simulink model "sampleModel103"  (R2023a)
settings: Solver=VariableStepAuto  StartTime=0.0  StopTime=10.0  RelTol=1e-3
undefined symbols (not defined in the file): DiscIntNeverNeededParam, Newton, Raphson
libraries: simulink x49, slpidlib x14
(part 1 of 3)
settings Model: Creator=TSMC  LastModifiedBy=TSMC

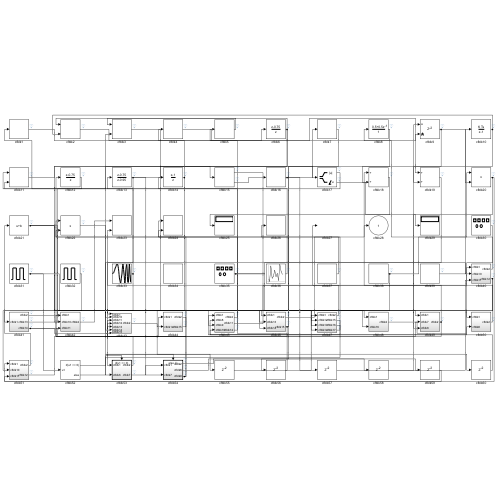
[thumbnail: Simulink's stored preview of the top-level diagram]
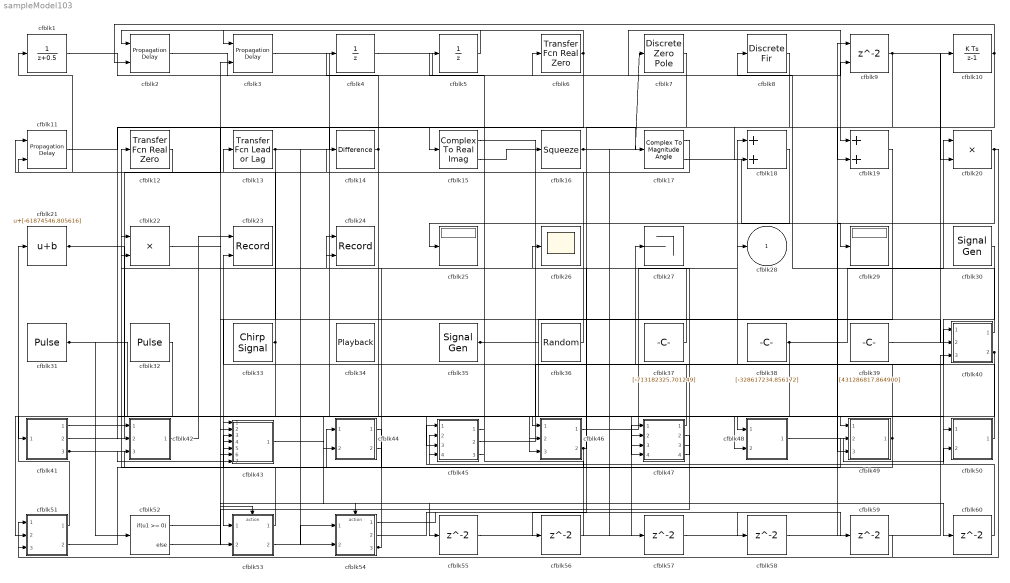
== system sampleModel103 ==
  cfblk1 : DiscreteTransferFcn  SampleTime=1
  cfblk10 : DiscreteIntegrator  ICPrevOutput=DiscIntNeverNeededParam  ICPrevScaledInput=DiscIntNeverNeededParam
  cfblk11 : PropagationDelay  SampleTime=1
  cfblk12 : simulink/Discrete/Transfer Fcn Real Zero  ZeroZ=0.75  ICPrevInput=0.0  DoSatur=off
  cfblk13 : simulink/Discrete/Transfer Fcn Lead or Lag  PoleZ=0.95  ZeroZ=0.75  ICPrevOutput=0.0  ICPrevInput=0.0  DoSatur=off
  cfblk14 : simulink/Discrete/Difference  ICPrevInput=0.0  OutMin=[]  OutMax=[]  OutDataTypeStr=Inherit: Inherit via back propagation  OutDataType=fixdt(1, 16)  OutScaling=2^-10  DoSatur=off
  cfblk15 : ComplexToRealImag
  cfblk16 : Squeeze
  cfblk17 : ComplexToMagnitudeAngle
  cfblk18 : Sum
  cfblk19 : Sum
  cfblk2 : PropagationDelay  SampleTime=1
  cfblk20 : Product
  cfblk21 : Bias  Bias=[-61874546.805616]  SaturateOnIntegerOverflow=off
  cfblk22 : Product  Inputs=**
  cfblk23 : Record  FileSettingsInternal="{\"entries\":[{\"content\":{\"excelSettings\":{\"content\":{},\"type\":\"Streamout.ExcelSettings\"}},\"type\":\"Streamout.FileSettingStorage\",\"uuid\":\"\"}],\"packageUris\":[\"http:\\/\\/schema.mathworks.com\\/mf0\\/streamout_blocks\\/R2020a\"],\"version\":\"1.0\"}"  Layout=[1 1]  SignalsInternal="{\"entries\":[{\"content\":{\"signals\":[{\"content\":{\"blockPath\":[],\"dimensions\":[1],\"domain\":\"\",\"lineColor\":\"#a2142f\",\"plots\":[1],\"port\":1,\"sid\":[\"\"],\"signalID\":5186,\"signalName\":\"cfblk42\"},\"type\":\"RecordBlkView.Signal\",\"uuid\":\"\"},{\"content\":{\"blockPath\":[],\"dimensions\":[1],\"domain\":\"\",\"lineColor\":\"#139fff\",\"plots\":[1],\"port\":2,\"sid\":[\"\"],\"signalID\":5190,\"signalName\":\"cfblk49\"},\"type\":\"RecordBlkView.Signal\",\"uuid\":\"\"}]},\"type\":\"RecordBlkView.InputSignals\",\"uuid\":\"\"}],\"packageUris\":[\"http:\\/\\/schema.mathworks.com\\/mf0\\/streamout_blocks\\/R2020a\"],\"version\":\"1.0\"}"  VisualizationBindings="{\"xyplotplugin\":{\"info\":[{\"series\":[{\"bindingParametersList\":[{\"parameter\":\"X-Axis\",\"signalID\":5186,\"signalName\":\"cfblk42\"},{\"parameter\":\"Y-Axis\",\"signalID\":5190,\"signalName\":\"cfblk49\"}],\"seriesID\":55035}],\"subplotID\":1}]}}"  CompatibilityTag=XY
  cfblk24 : Record  FileSettingsInternal="{\"entries\":[{\"content\":{\"excelSettings\":{\"content\":{},\"type\":\"Streamout.ExcelSettings\"}},\"type\":\"Streamout.FileSettingStorage\",\"uuid\":\"\"}],\"packageUris\":[\"http:\\/\\/schema.mathworks.com\\/mf0\\/streamout_blocks\\/R2020a\"],\"version\":\"1.0\"}"  Layout=[1 1]  SignalsInternal="{\"entries\":[{\"content\":{\"signals\":[{\"content\":{\"blockPath\":[],\"dimensions\":[1],\"domain\":\"\",\"lineColor\":\"#a2142f\",\"plots\":[1],\"port\":1,\"sid\":[\"\"],\"signalID\":5194,\"signalName\":\"cfblk46:2\"},\"type\":\"RecordBlkView.Signal\",\"uuid\":\"\"},{\"content\":{\"blockPath\":[],\"dimensions\":[1],\"domain\":\"\",\"lineColor\":\"#139fff\",\"plots\":[1],\"port\":2,\"sid\":[\"\"],\"signalID\":5198,\"signalName\":\"cfblk37\"},\"type\":\"RecordBlkView.Signal\",\"uuid\":\"\"}]},\"type\":\"RecordBlkView.InputSignals\",\"uuid\":\"\"}],\"packageUris\":[\"http:\\/\\/schema.mathworks.com\\/mf0\\/streamout_blocks\\/R2020a\"],\"version\":\"1.0\"}"  VisualizationBindings="{\"xyplotplugin\":{\"info\":[{\"series\":[{\"bindingParametersList\":[{\"parameter\":\"X-Axis\",\"signalID\":5194,\"signalName\":\"cfblk46:2\"},{\"parameter\":\"Y-Axis\",\"signalID\":5198,\"signalName\":\"cfblk37\"}],\"seriesID\":45192}],\"subplotID\":1}]}}"  CompatibilityTag=XY
  cfblk25 : Display
  cfblk26 : Scope
  cfblk27 : Terminator
  cfblk29 : Display
  cfblk3 : PropagationDelay  SampleTime=1
  cfblk30 : SignalGenerator  WaveForm=sawtooth  Amplitude=[-997237274.196196]
  cfblk31 : DiscretePulseGenerator  PulseType=Time based  Amplitude=[-749232423.157370]  Period=[74696247.311813]  PulseWidth=5  PhaseDelay=[8.000000]
  cfblk32 : DiscretePulseGenerator  PulseType=Time based  Amplitude=[-196614615.900972]  Period=[15763149.979397]  PulseWidth=5  PhaseDelay=[2.000000]
  cfblk33 : simulink/Sources/Chirp Signal  f1=[865246952.903750]  T=[-111365965.632688]  f2=[-44710959.948198]
  cfblk34 : Playback  NumPorts=0  PartName=eaea7638-26f9-48da-bb3d-fef66314ee33
  cfblk35 : SignalGenerator  Amplitude=[-962831918.348630]  Units=rad/sec
  cfblk36 : UniformRandomNumber  Minimum=[-5524023803.668765]  Maximum=[1433073100.815679]  Seed=[27130388.000000]  SampleTime=0.1
  cfblk37 : Constant  Value=[-713182325.701249]  SampleTime=1
  cfblk38 : Constant  Value=[-328617234.856172]  SampleTime=1
  cfblk39 : Constant  Value=[431286817.864900]  SampleTime=1
  cfblk4 : UnitDelay  HasFrameUpgradeWarning=on
  cfblk40 : Subsystem
  cfblk41 : Subsystem
  cfblk42 : Subsystem
  cfblk43 : Subsystem
  cfblk44 : Subsystem
  cfblk45 : Subsystem
  cfblk46 : Subsystem
  cfblk47 : Subsystem
  cfblk48 : Subsystem
  cfblk49 : Subsystem
  cfblk5 : UnitDelay  HasFrameUpgradeWarning=on
  cfblk50 : Subsystem
  cfblk51 : Subsystem
  cfblk52 : If  IfExpression=u1 >= 0  SampleTime=1
  cfblk53 : Subsystem  TreatAsAtomicUnit=on
  cfblk54 : Subsystem  TreatAsAtomicUnit=on
  cfblk{55..60} (6 alike) : Delay  SampleTime=1
  cfblk6 : simulink/Discrete/Transfer Fcn Real Zero  ZeroZ=0.75  ICPrevInput=0.0  DoSatur=off
  cfblk7 : DiscreteZeroPole  Poles=[0 0.5]  Gain=1
  cfblk8 : DiscreteFir  SampleTime=1
  cfblk9 : Delay  ShowEnablePort=on  SampleTime=1
      settings: InputPortMap=u0,e6
  cfblk28 : Outport
  wires:
  cfblk38/1 -> cfblk20/1, cfblk47/2(cfblk12)
  cfblk42/1(cfblk2) -> cfblk23/1
  cfblk17/1 -> cfblk13/1
  cfblk13/1 -> cfblk15/1, cfblk54/2(cfblk7), cfblk43/6(cfblk14)
  cfblk6/1 -> cfblk3/1, cfblk42/2(cfblk10), cfblk43/2(cfblk10)
  cfblk16/1 -> cfblk7/1, cfblk57/1
  cfblk39/1 -> cfblk10/1
  cfblk30/1 -> cfblk45/2(cfblk8)
  cfblk51/1(cfblk2) -> cfblk21/1
  cfblk15/1 -> cfblk48/1(cfblk1)
  cfblk44/1(cfblk2) -> cfblk12/1
  cfblk35/1 -> cfblk49/1(cfblk1), cfblk40/2(cfblk10)
  cfblk9/1 -> cfblk20/2, cfblk19/2
  cfblk11/1 -> cfblk17/1
  cfblk31/1 -> cfblk52/1, cfblk46/2(cfblk13)
  cfblk3/1 -> cfblk48/2(cfblk16)
  cfblk47/1(cfblk2) -> cfblk27/1
  cfblk46/1(cfblk2) -> cfblk18/1
  cfblk5/1 -> cfblk2/1
  cfblk4/1 -> cfblk19/1
  cfblk41/1(cfblk2) -> cfblk45/3(cfblk9)
  cfblk46/2(cfblk15) -> cfblk24/1, cfblk43/5(cfblk13)
  cfblk10/1 -> cfblk2/2, cfblk46/1(cfblk1)
  cfblk20/1 -> cfblk51/1(cfblk1), cfblk49/3(cfblk8)
  cfblk47/2(cfblk15) -> cfblk45/4(cfblk10)
  cfblk21/1 -> cfblk50/1(cfblk1), cfblk47/3(cfblk13), cfblk47/4(cfblk14)
  cfblk50/1(cfblk2) -> cfblk28/1
  cfblk19/1 -> cfblk53/1(cfblk1)
  cfblk36/1 -> cfblk14/1
  cfblk40/1(cfblk2) -> cfblk8/1
  cfblk37/1 -> cfblk24/2
  cfblk47/3(cfblk16) -> cfblk53/2(cfblk6)
  cfblk47/4(cfblk17) -> cfblk26/1
  cfblk14/1 -> cfblk4/1, cfblk43/7(cfblk15)
  cfblk33/1 -> cfblk1/1, cfblk41/1(cfblk1)
  cfblk2/1 -> cfblk6/1
  cfblk44/2(cfblk15) -> cfblk43/1(cfblk1)
  cfblk41/2(cfblk13) -> cfblk3/2
  cfblk12/1 -> cfblk11/2
  cfblk15/2 -> cfblk16/1
  cfblk51/2(cfblk12) -> cfblk44/1(cfblk1)
  cfblk17/2 -> cfblk29/1
  cfblk32/1 -> cfblk51/2(cfblk10)
  cfblk45/1(cfblk2) -> cfblk5/1
  cfblk18/1 -> cfblk25/1
  cfblk49/1(cfblk2) -> cfblk23/2, cfblk42/3(cfblk11)
  cfblk48/1(cfblk2) -> cfblk50/2(cfblk8)
  cfblk40/2(cfblk12) -> cfblk44/2(cfblk14), cfblk46/3(cfblk14)
  cfblk8/1 -> cfblk18/2
  cfblk53/1(cfblk2) -> cfblk42/1(cfblk1)
  cfblk45/2(cfblk11) -> cfblk40/1(cfblk1)
  cfblk53/2(cfblk7) -> cfblk54/1(cfblk1)
  cfblk45/3(cfblk12) -> cfblk22/1
  cfblk1/1 -> cfblk9/2
  cfblk54/3(cfblk9) -> cfblk22/2, cfblk43/4(cfblk12)
  cfblk41/3(cfblk14) -> cfblk49/2(cfblk7), cfblk43/3(cfblk11)
  cfblk52/1 -> cfblk53/Action
  cfblk52/2 -> cfblk54/Action
  cfblk43/1(cfblk2) -> cfblk55/1
  cfblk55/1 -> cfblk47/1(cfblk1)
  cfblk7/1 -> cfblk56/1
  cfblk56/1 -> cfblk11/1
  cfblk57/1 -> cfblk40/3(cfblk11)
  cfblk54/1(cfblk2) -> cfblk58/1
  cfblk58/1 -> cfblk9/1
  cfblk54/2(cfblk8) -> cfblk59/1
  cfblk59/1 -> cfblk51/3(cfblk11)
  cfblk22/1 -> cfblk60/1
  cfblk60/1 -> cfblk45/1(cfblk1)

== system sampleModel103/cfblk40 ==
  cfblk1 : Inport
  cfblk10 : Inport  Port=2
  cfblk11 : Inport  Port=3
  cfblk3 : simulink/Discrete/Tapped Delay  vinit=0.0  samptime=-1  NumDelays=1  DelayOrder=Oldest  includeCurrent=off
  cfblk4 : Sum  Inputs=+
  cfblk5 : Math  Operator=conj
  cfblk6 : Sqrt  Operator=rSqrt  AlgorithmType=Newton-Raphson
  cfblk7 : Constant  Value=[694458684.755067]  SampleTime=1
  cfblk8 : Subsystem
  cfblk9 : Subsystem
  cfblk2 : Outport
  cfblk12 : Outport  Port=2
  wires:
  cfblk10/1 -> cfblk3/1
  cfblk11/1 -> cfblk12/1
  cfblk7/1 -> cfblk5/1
  cfblk9/1(cfblk2) -> cfblk2/1
  cfblk3/1 -> cfblk6/1
  cfblk4/1 -> cfblk8/1(cfblk1), cfblk8/3(cfblk12)
  cfblk6/1 -> cfblk9/1(cfblk1)
  cfblk1/1 -> cfblk4/1
  cfblk5/1 -> cfblk8/2(cfblk11)
  cfblk8/1(cfblk2) -> cfblk9/2(cfblk8)

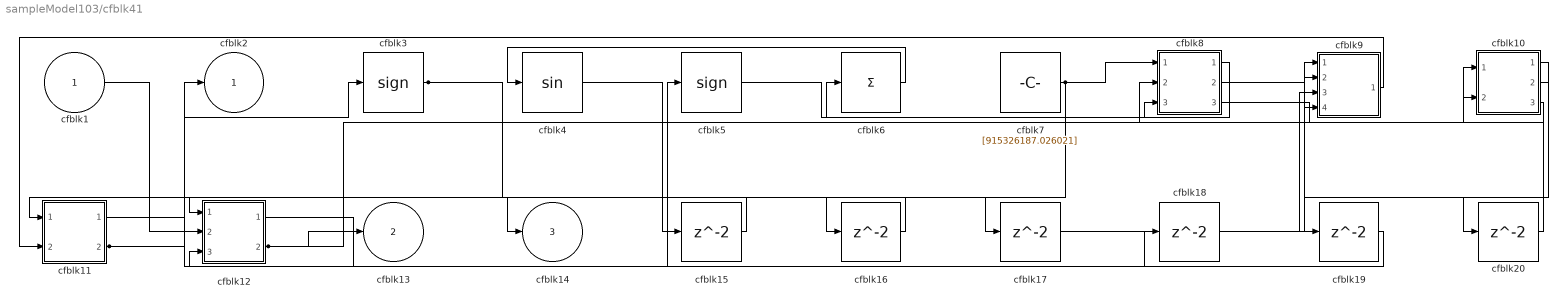
== system sampleModel103/cfblk41 ==
  cfblk1 : Inport
  cfblk10 : Subsystem
  cfblk11 : Subsystem
  cfblk12 : Subsystem
  cfblk{15..20} (6 alike) : Delay  SampleTime=1
  cfblk3 : Signum
  cfblk4 : Trigonometry
  cfblk5 : Signum
  cfblk6 : Sum  Inputs=+
  cfblk7 : Constant  Value=[915326187.026021]  SampleTime=1
  cfblk8 : Subsystem
  cfblk9 : Subsystem
  cfblk2 : Outport
  cfblk13 : Outport  Port=2
  cfblk14 : Outport  Port=3
  wires:
  cfblk6/1 -> cfblk4/1
  cfblk8/1(cfblk2) -> cfblk6/1
  cfblk7/1 -> cfblk8/1(cfblk1), cfblk14/1
  cfblk1/1 -> cfblk12/2(cfblk10)
  cfblk12/1(cfblk2) -> cfblk5/1
  cfblk8/2(cfblk16) -> cfblk9/1(cfblk1)
  cfblk3/1 -> cfblk16/1, cfblk17/1
  cfblk8/3(cfblk17) -> cfblk10/1(cfblk1)
  cfblk9/1(cfblk2) -> cfblk11/2(cfblk6)
  cfblk11/1(cfblk2) -> cfblk2/1
  cfblk12/2(cfblk12) -> cfblk13/1, cfblk10/2(cfblk14)
  cfblk5/1 -> cfblk8/3(cfblk15)
  cfblk11/2(cfblk7) -> cfblk3/1, cfblk18/1
  cfblk10/3(cfblk16) -> cfblk9/2(cfblk6)
  cfblk4/1 -> cfblk15/1
  cfblk15/1 -> cfblk12/1(cfblk1)
  cfblk16/1 -> cfblk11/1(cfblk1)
  cfblk17/1 -> cfblk9/4(cfblk8)
  cfblk18/1 -> cfblk9/3(cfblk7)
  cfblk10/1(cfblk2) -> cfblk19/1
  cfblk19/1 -> cfblk12/3(cfblk11)
  cfblk10/2(cfblk15) -> cfblk20/1
  cfblk20/1 -> cfblk8/2(cfblk14)

== system sampleModel103/cfblk42 ==
  cfblk1 : Inport
  cfblk10 : Inport  Port=2
  cfblk11 : Inport  Port=3
  cfblk12 : Delay  SampleTime=1
  cfblk13 : Delay  SampleTime=1
  cfblk3 : Delay  ShowEnablePort=on  SampleTime=1
      settings: InputPortMap=u0,e6
  cfblk4 : Product  Inputs=*
  cfblk5 : Product  Inputs=**
  cfblk6 : Sum  Inputs=+-
  cfblk7 : Subsystem
  cfblk8 : Subsystem
  cfblk9 : Subsystem
  cfblk2 : Outport
  wires:
  cfblk3/1 -> cfblk8/1(cfblk1)
  cfblk10/1 -> cfblk7/1(cfblk1)
  cfblk11/1 -> cfblk7/2(cfblk7)
  cfblk6/1 -> cfblk4/1
  cfblk7/1(cfblk2) -> cfblk5/1
  cfblk7/2(cfblk8) -> cfblk3/1
  cfblk1/1 -> cfblk2/1
  cfblk4/1 -> cfblk5/2
  cfblk8/1(cfblk2) -> cfblk9/2(cfblk5)
  cfblk9/2(cfblk6) -> cfblk6/1
  cfblk9/3(cfblk7) -> cfblk6/2
  cfblk9/1(cfblk2) -> cfblk12/1
  cfblk12/1 -> cfblk3/2
  cfblk5/1 -> cfblk13/1
  cfblk13/1 -> cfblk9/1(cfblk1)

== system sampleModel103/cfblk43 ==
  cfblk1 : Inport
  cfblk10 : Inport  Port=2
  cfblk11 : Inport  Port=3
  cfblk12 : Inport  Port=4
  cfblk13 : Inport  Port=5
  cfblk14 : Inport  Port=6
  cfblk15 : Inport  Port=7
  cfblk3 : simulink/Discrete/Transfer Fcn Real Zero  ZeroZ=0.75  ICPrevInput=0.0  DoSatur=off
  cfblk4 : slpidlib/PID Controller  Controller=PID  Form=Parallel  TimeDomain=Discrete-time  UseExternalTs=off  SampleTime=1  IntegratorMethod=Forward Euler  FilterMethod=Forward Euler  ControllerParametersSource=internal  P=1  I=1  UseKiTs=off  D=0  N=100  UseFilter=on  TunerSelectOption=Transfer Function Based (PID Tuner App)  InitialConditionSource=internal  InitialConditionForIntegrator=0  InitialConditionForFilter=0  DifferentiatorICPrevScaledInput=0  ExternalReset=none  TrackingMode=off  Kt=1  LimitOutput=off  SatLimitsSource=internal  UpperSaturationLimit=inf  LowerSaturationLimit=-inf  LinearizeAsGain=off  AntiWindupMode=none  Kb=1  LimitIntegrator=off  UpperIntegratorSaturationLimit=inf  LowerIntegratorSaturationLimit=-inf  POutMin=[]  POutMax=[]  IOutMin=[]  IOutMax=[]  DOutMin=[]  DOutMax=[]  NOutMin=[]  NOutMax=[]  SumOutMin=[]  SumOutMax=[]  SaturationOutMin=[]  SaturationOutMax=[]  PParamMin=[]  PParamMax=[]  IParamMin=[]  IParamMax=[]  DParamMin=[]  DParamMax=[]  NParamMin=[]  NParamMax=[]  KbParamMin=[]  KbParamMax=[]  KtParamMin=[]  KtParamMax=[]  KbOutMin=[]  KbOutMax=[]  KtOutMin=[]  KtOutMax=[]  IntegratorOutMin=[]  IntegratorOutMax=[]  FilterOutMin=[]  FilterOutMax=[]  SumI1OutMin=[]  SumI1OutMax=[]  SumI2OutMin=[]  SumI2OutMax=[]  SumI3OutMin=[]  SumI3OutMax=[]  SumI4OutMin=[]  SumI4OutMax=[]  SumDOutMin=[]  SumDOutMax=[]  DifferentiatorOutMin=[]  DifferentiatorOutMax=[]  FilterDiffOutCoefMin=[]  FilterDiffOutCoefMax=[]  ReciprocalOutMin=[]  ReciprocalOutMax=[]  SumDenOutMin=[]  SumDenOutMax=[]  SumNumOutMin=[]  SumNumOutMax=[]  DivideOutMin=[]  DivideOutMax=[]  UdiffTsProdOutMin=[]  UdiffTsProdOutMax=[]  NTsProdOutMin=[]  NTsProdOutMax=[]  UintegralTsProdOutMin=[]  UintegralTsProdOutMax=[]  UngainTsProdOutMin=[]  UngainTsProdOutMax=[]  ClampingZeroOutDataTypeStr=Inherit: Inherit via back propagation  ClampingZeroOutMin=[]  ClampingZeroOutMax=[]  FilterDenConstantOutDataTypeStr=Inherit: Inherit via back propagation  FilterDenConstantOutMin=[]  FilterDenConstantOutMax=[]  PCopyOutDataTypeStr=Inherit: Inherit via back propagation  PCopyOutMin=[]  PCopyOutMax=[]  NCopyOutDataTypeStr=Inherit: Inherit via back propagation  NCopyOutMin=[]  NCopyOutMax=[]  IntegratorContinuousStateAttributes=''  IntegratorStateMustResolveToSignalObject=off  IntegratorRTWStateStorageClass=Auto  FilterContinuousStateAttributes=''  FilterStateMustResolveToSignalObject=off  FilterRTWStateStorageClass=Auto  ParallelPVariant=InternalParameters  IdealPVariant=Disabled  IVariant=InternalParameters  DVariant=InternalParameters  IntegratorVariant=Discrete  SatVariant=Disabled  AWVariant=Passthrough  PCopyVariant=Disabled  TRVariant=Disabled  FdbkBlocksVariant=Forward  IdealPFdbkVariant=Disabled  SatFdbkVariant=Disabled  DerivativeFilterVariant=ForwardEulerFilter  NVariant=InternalParameters  NCopyVariant=Disabled  FilterICVariant=InternalICsFilter  IntegratorICVariant=InternalICs  ExternalResetVariant=Disabled  TRSumVariant=Passthrough  SumFdbkVariant=Disabled  SumVariant=Sum_PID  TsampFilterVariant=InternalTs  TsampNgainVariant=Passthrough  TsampIntegralVariant=Disabled_SignalSpec  ExternalSaturationOutDataTypeStr=Inherit: Same as second input
      settings: LibrarySourceBlock=simulink/Discrete/Discrete PID Controller
  cfblk5 : simulink/Math Operations/Slider Gain  gain=1  low=0  high=2
  cfblk6 : Sqrt  Operator=rSqrt  AlgorithmType=Newton-Raphson
  cfblk7 : simulink/Math Operations/MinMax Running Resettable  Function=min  vinit=0.0
  cfblk8 : Subsystem
  cfblk9 : Subsystem
  cfblk2 : Outport
  wires:
  cfblk1/1 -> cfblk7/1
  cfblk6/1 -> cfblk4/1
  cfblk3/1 -> cfblk2/1
  cfblk11/1 -> cfblk8/1(cfblk1)
  cfblk7/1 -> cfblk3/1
  cfblk10/1 -> cfblk6/1
  cfblk4/1 -> cfblk9/1(cfblk1)
  cfblk9/1(cfblk2) -> cfblk7/2
  cfblk8/1(cfblk2) -> cfblk9/2(cfblk14)
  cfblk5/1 -> cfblk9/3(cfblk15)
  cfblk14/1 -> cfblk5/1

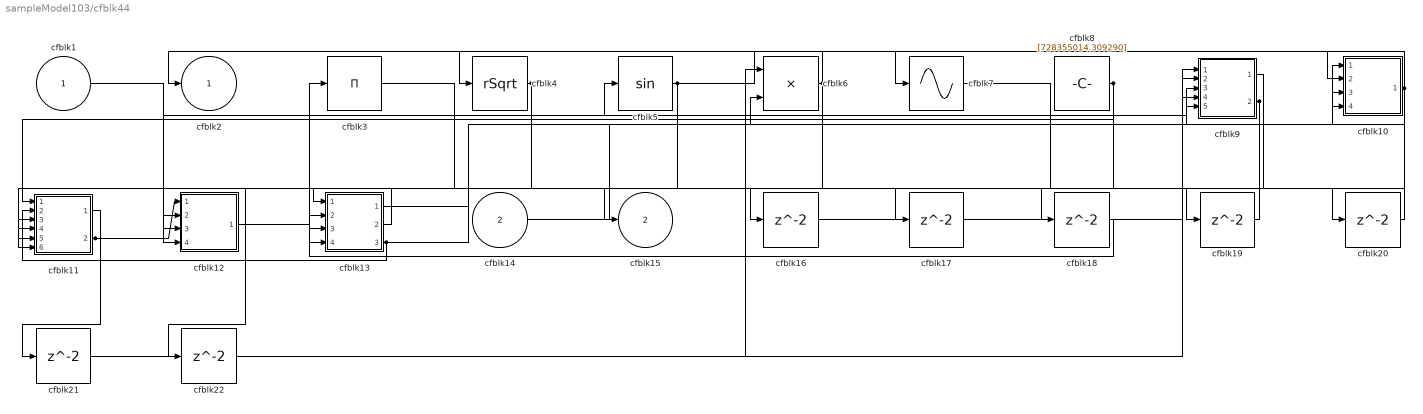
== system sampleModel103/cfblk44 ==
  cfblk1 : Inport
  cfblk14 : Inport  Port=2
  cfblk10 : Subsystem
  cfblk11 : Subsystem
  cfblk12 : Subsystem
  cfblk13 : Subsystem
  cfblk{16..22} (7 alike) : Delay  SampleTime=1
  cfblk3 : Product  Inputs=*
  cfblk4 : Sqrt  Operator=rSqrt  AlgorithmType=Newton-Raphson
  cfblk5 : Trigonometry
  cfblk6 : Product
  cfblk7 : Sin  TimeSource=Use external signal  SampleTime=0
  cfblk8 : Constant  Value=[728355014.309290]  SampleTime=1
  cfblk9 : Subsystem
  cfblk2 : Outport
  cfblk15 : Outport  Port=2
  wires:
  cfblk14/1 -> cfblk10/1(cfblk1)
  cfblk10/1(cfblk2) -> cfblk2/1, cfblk7/1, cfblk18/1, cfblk20/1
  cfblk8/1 -> cfblk11/1(cfblk1), cfblk11/5(cfblk14)
  cfblk9/1(cfblk2) -> cfblk15/1
  cfblk11/2(cfblk16) -> cfblk12/1(cfblk1), cfblk5/1
  cfblk6/1 -> cfblk4/1, cfblk11/6(cfblk15)
  cfblk9/2(cfblk16) -> cfblk13/1(cfblk1), cfblk6/2, cfblk12/4(cfblk7), cfblk11/3(cfblk12)
  cfblk5/1 -> cfblk10/2(cfblk11), cfblk12/3(cfblk6), cfblk10/4(cfblk13)
  cfblk1/1 -> cfblk9/3(cfblk13)
  cfblk12/1(cfblk2) -> cfblk3/1
  cfblk13/2(cfblk10) -> cfblk12/2(cfblk5)
  cfblk4/1 -> cfblk13/4(cfblk9), cfblk11/4(cfblk13), cfblk22/1
  cfblk13/3(cfblk11) -> cfblk10/3(cfblk12), cfblk11/2(cfblk11)
  cfblk13/1(cfblk2) -> cfblk16/1
  cfblk16/1 -> cfblk9/2(cfblk12)
  cfblk3/1 -> cfblk17/1
  cfblk17/1 -> cfblk9/4(cfblk14)
  cfblk18/1 -> cfblk13/3(cfblk8)
  cfblk7/1 -> cfblk19/1
  cfblk19/1 -> cfblk13/2(cfblk7)
  cfblk20/1 -> cfblk9/5(cfblk15)
  cfblk11/1(cfblk2) -> cfblk21/1
  cfblk21/1 -> cfblk9/1(cfblk1)
  cfblk22/1 -> cfblk6/1

== system sampleModel103/cfblk45 ==
  cfblk1 : Inport
  cfblk8 : Inport  Port=2
  cfblk9 : Inport  Port=3
  cfblk10 : Inport  Port=4
  cfblk13 : Delay  SampleTime=1
  cfblk14 : Delay  SampleTime=1
  cfblk15 : Delay  SampleTime=1
  cfblk3 : slpidlib/PID Controller (2DOF)  Controller=PID  Form=Parallel  TimeDomain=Discrete-time  UseExternalTs=off  SampleTime=1  IntegratorMethod=Forward Euler  FilterMethod=Forward Euler  ControllerParametersSource=internal  P=1  I=1  UseKiTs=off  D=0  N=100  UseFilter=on  b=1  c=1  TunerSelectOption=Transfer Function Based (PID Tuner App)  InitialConditionSource=internal  InitialConditionForIntegrator=0  InitialConditionForFilter=0  DifferentiatorICPrevScaledInput=0  ExternalReset=none  TrackingMode=off  Kt=1  LimitOutput=off  SatLimitsSource=internal  UpperSaturationLimit=inf  LowerSaturationLimit=-inf  LinearizeAsGain=off  AntiWindupMode=none  Kb=1  LimitIntegrator=off  UpperIntegratorSaturationLimit=inf  LowerIntegratorSaturationLimit=-inf  POutMin=[]  POutMax=[]  IOutMin=[]  IOutMax=[]  DOutMin=[]  DOutMax=[]  NOutMin=[]  NOutMax=[]  bOutMin=[]  bOutMax=[]  cOutMin=[]  cOutMax=[]  SumOutMin=[]  SumOutMax=[]  SaturationOutMin=[]  SaturationOutMax=[]  PParamMin=[]  PParamMax=[]  IParamMin=[]  IParamMax=[]  DParamMin=[]  DParamMax=[]  NParamMin=[]  NParamMax=[]  bParamMin=[]  bParamMax=[]  cParamMin=[]  cParamMax=[]  KbParamMin=[]  KbParamMax=[]  KtParamMin=[]  KtParamMax=[]  KbOutMin=[]  KbOutMax=[]  KtOutMin=[]  KtOutMax=[]  IntegratorOutMin=[]  IntegratorOutMax=[]  FilterOutMin=[]  FilterOutMax=[]  SumI1OutMin=[]  SumI1OutMax=[]  SumI2OutMin=[]  SumI2OutMax=[]  SumI3OutMin=[]  SumI3OutMax=[]  SumI4OutMin=[]  SumI4OutMax=[]  SumDOutMin=[]  SumDOutMax=[]  Sum1OutMin=[]  Sum1OutMax=[]  Sum2OutMin=[]  Sum2OutMax=[]  Sum3OutMin=[]  Sum3OutMax=[]  DifferentiatorOutMin=[]  DifferentiatorOutMax=[]  FilterDiffOutCoefMin=[]  FilterDiffOutCoefMax=[]  ReciprocalOutMin=[]  ReciprocalOutMax=[]  SumDenOutMin=[]  SumDenOutMax=[]  SumNumOutMin=[]  SumNumOutMax=[]  DivideOutMin=[]  DivideOutMax=[]  UdiffTsProdOutMin=[]  UdiffTsProdOutMax=[]  NTsProdOutMin=[]  NTsProdOutMax=[]  UintegralTsProdOutMin=[]  UintegralTsProdOutMax=[]  UngainTsProdOutMin=[]  UngainTsProdOutMax=[]  ClampingZeroOutDataTypeStr=Inherit: Inherit via back propagation  ClampingZeroOutMin=[]  ClampingZeroOutMax=[]  FilterDenConstantOutDataTypeStr=Inherit: Inherit via back propagation  FilterDenConstantOutMin=[]  FilterDenConstantOutMax=[]  PCopyOutDataTypeStr=Inherit: Inherit via back propagation  PCopyOutMin=[]  PCopyOutMax=[]  NCopyOutDataTypeStr=Inherit: Inherit via back propagation  NCopyOutMin=[]  NCopyOutMax=[]  IntegratorContinuousStateAttributes=''  IntegratorStateMustResolveToSignalObject=off  IntegratorRTWStateStorageClass=Auto  FilterContinuousStateAttributes=''  FilterStateMustResolveToSignalObject=off  FilterRTWStateStorageClass=Auto  ParallelPVariant=InternalParameters  IdealPVariant=Disabled  IVariant=InternalParameters  DVariant=InternalParameters  bVariant=InternalParameters  cVariant=InternalParameters  IntegratorVariant=Discrete  SatVariant=Disabled  AWVariant=Passthrough  PCopyVariant=Disabled  TRVariant=Disabled  FdbkBlocksVariant=Forward  IdealPFdbkVariant=Disabled  SatFdbkVariant=Disabled  DerivativeFilterVariant=ForwardEulerFilter  NVariant=InternalParameters  NCopyVariant=Disabled  FilterICVariant=InternalICsFilter  IntegratorICVariant=InternalICs  ExternalResetVariant=Disabled  TRSumVariant=Passthrough  SumFdbkVariant=Disabled  SumVariant=Sum_PID  TsampFilterVariant=InternalTs  TsampNgainVariant=Passthrough  TsampIntegralVariant=Disabled_SignalSpec  ExternalSaturationOutDataTypeStr=Inherit: Same as second input
      settings: LibrarySourceBlock=simulink/Discrete/Discrete PID Controller (2DOF)
  cfblk4 : Sum  Inputs=--
  cfblk5 : Subsystem
  cfblk6 : Subsystem
  cfblk7 : Subsystem
  cfblk2 : Outport
  cfblk11 : Outport  Port=2
  cfblk12 : Outport  Port=3
  wires:
  cfblk8/1 -> cfblk11/1
  cfblk5/1(cfblk2) -> cfblk2/1
  cfblk9/1 -> cfblk4/1
  cfblk10/1 -> cfblk3/1
  cfblk6/1(cfblk2) -> cfblk12/1
  cfblk1/1 -> cfblk5/1(cfblk1)
  cfblk7/1(cfblk2) -> cfblk3/2
  cfblk7/2(cfblk17) -> cfblk4/2
  cfblk6/2(cfblk7) -> cfblk7/1(cfblk1)
  cfblk5/2(cfblk13) -> cfblk6/1(cfblk1)
  cfblk5/3(cfblk14) -> cfblk7/3(cfblk16)
  cfblk3/1 -> cfblk13/1
  cfblk13/1 -> cfblk6/2(cfblk6)
  cfblk4/1 -> cfblk14/1
  cfblk14/1 -> cfblk7/2(cfblk15)
  cfblk6/3(cfblk8) -> cfblk15/1
  cfblk15/1 -> cfblk5/2(cfblk12)

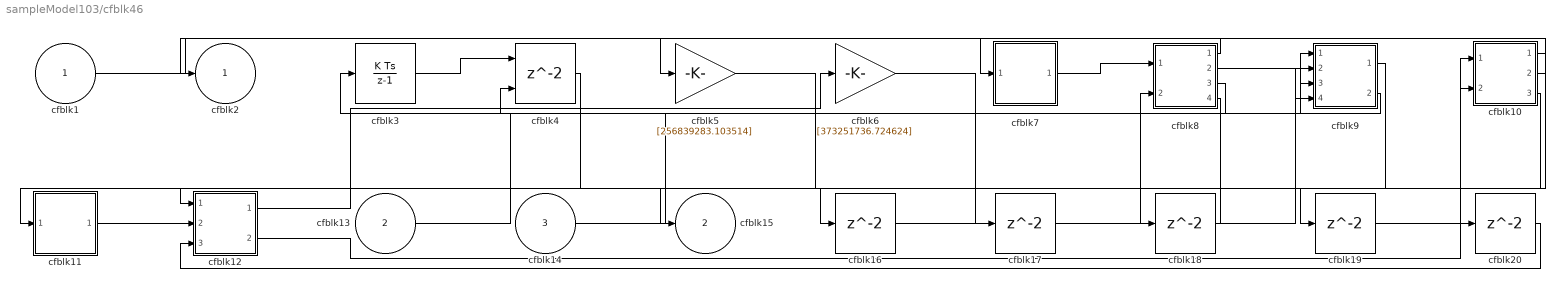
== system sampleModel103/cfblk46 ==
  cfblk1 : Inport
  cfblk13 : Inport  Port=2
  cfblk14 : Inport  Port=3
  cfblk10 : Subsystem
  cfblk11 : Subsystem
  cfblk12 : Subsystem
  cfblk{16..20} (5 alike) : Delay  SampleTime=1
  cfblk3 : DiscreteIntegrator  ICPrevOutput=DiscIntNeverNeededParam  ICPrevScaledInput=DiscIntNeverNeededParam
  cfblk4 : Delay  ShowEnablePort=on  SampleTime=1
      settings: InputPortMap=u0,e6
  cfblk5 : Gain  Gain=[256839283.103514]
  cfblk6 : Gain  Gain=[373251736.724624]
  cfblk7 : Subsystem
  cfblk8 : Subsystem
  cfblk9 : Subsystem
  cfblk2 : Outport
  cfblk15 : Outport  Port=2
  wires:
  cfblk12/1(cfblk2) -> cfblk6/1
  cfblk1/1 -> cfblk7/1(cfblk1)
  cfblk12/2(cfblk11) -> cfblk10/1(cfblk1)
  cfblk3/1 -> cfblk4/1
  cfblk7/1(cfblk2) -> cfblk8/1(cfblk1)
  cfblk4/1 -> cfblk11/1(cfblk1)
  cfblk13/1 -> cfblk9/1(cfblk1)
  cfblk14/1 -> cfblk9/3(cfblk11)
  cfblk9/2(cfblk13) -> cfblk4/2
  cfblk8/1(cfblk2) -> cfblk2/1
  cfblk8/2(cfblk9) -> cfblk9/4(cfblk12)
  cfblk10/2(cfblk15) -> cfblk5/1
  cfblk11/1(cfblk2) -> cfblk12/2(cfblk9)
  cfblk8/3(cfblk10) -> cfblk3/1
  cfblk8/4(cfblk11) -> cfblk15/1
  cfblk9/1(cfblk2) -> cfblk16/1
  cfblk16/1 -> cfblk8/2(cfblk8)
  cfblk6/1 -> cfblk17/1
  cfblk17/1 -> cfblk9/2(cfblk10)
  cfblk10/1(cfblk2) -> cfblk18/1
  cfblk18/1 -> cfblk12/1(cfblk1)
  cfblk5/1 -> cfblk19/1
  cfblk19/1 -> cfblk10/2(cfblk14)
  cfblk10/3(cfblk16) -> cfblk20/1
  cfblk20/1 -> cfblk12/3(cfblk10)

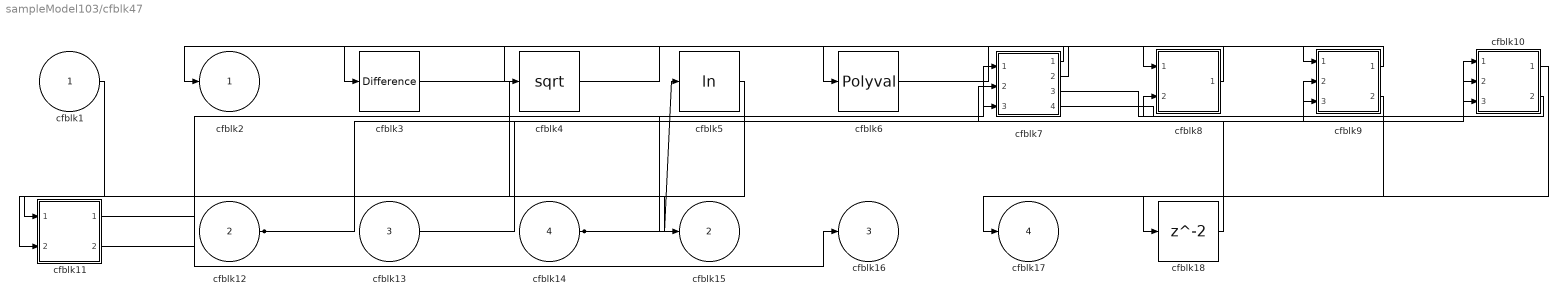
== system sampleModel103/cfblk47 ==
  cfblk1 : Inport
  cfblk12 : Inport  Port=2
  cfblk13 : Inport  Port=3
  cfblk14 : Inport  Port=4
  cfblk10 : Subsystem
  cfblk11 : Subsystem
  cfblk18 : Delay  SampleTime=1
  cfblk3 : simulink/Discrete/Difference  ICPrevInput=0.0  OutMin=[]  OutMax=[]  OutDataTypeStr=Inherit: Inherit via back propagation  OutDataType=fixdt(1, 16)  OutScaling=2^-10  DoSatur=off
  cfblk4 : Sqrt
  cfblk5 : Math  Operator=log
  cfblk6 : Polyval  Coefs=[ +2.081618890e-019, -1.441693666e-014, +4.719686976e-010, -8.536869453e-006, +1.621573104e-001, -8.087801117e+001 ]
  cfblk7 : Subsystem
  cfblk8 : Subsystem
  cfblk9 : Subsystem
  cfblk2 : Outport
  cfblk15 : Outport  Port=2
  cfblk16 : Outport  Port=3
  cfblk17 : Outport  Port=4
  wires:
  cfblk13/1 -> cfblk10/1(cfblk1)
  cfblk14/1 -> cfblk5/1, cfblk7/3(cfblk13)
  cfblk11/1(cfblk2) -> cfblk16/1
  cfblk7/1(cfblk2) -> cfblk3/1
  cfblk6/1 -> cfblk9/1(cfblk1)
  cfblk4/1 -> cfblk8/1(cfblk1)
  cfblk3/1 -> cfblk15/1
  cfblk10/1(cfblk2) -> cfblk17/1
  cfblk10/2(cfblk13) -> cfblk8/2(cfblk12)
  cfblk12/1 -> cfblk9/2(cfblk6), cfblk10/3(cfblk12)
  cfblk1/1 -> cfblk11/1(cfblk1)
  cfblk11/2(cfblk7) -> cfblk7/1(cfblk1)
  cfblk5/1 -> cfblk11/2(cfblk6)
  cfblk7/2(cfblk14) -> cfblk6/1
  cfblk8/1(cfblk2) -> cfblk2/1
  cfblk9/1(cfblk2) -> cfblk4/1
  cfblk7/3(cfblk15) -> cfblk9/3(cfblk7)
  cfblk7/4(cfblk16) -> cfblk10/2(cfblk11)
  cfblk9/2(cfblk8) -> cfblk18/1
  cfblk18/1 -> cfblk7/2(cfblk12)

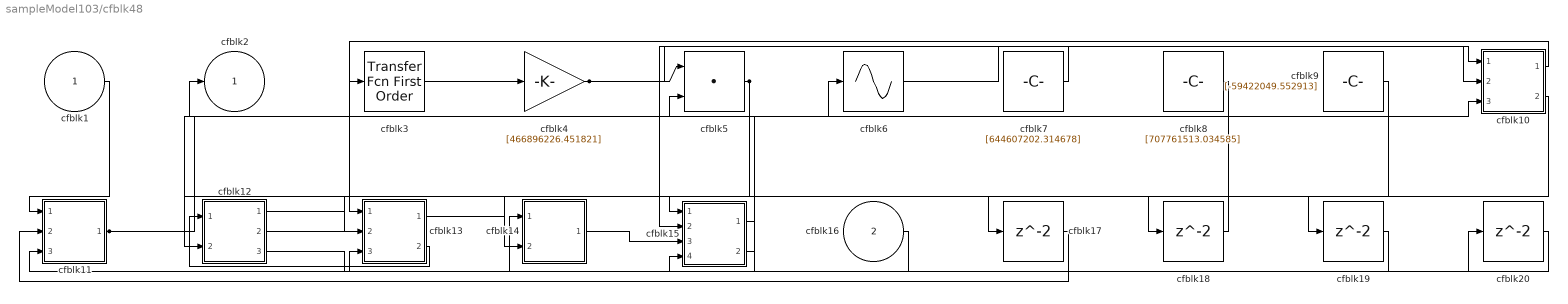
== system sampleModel103/cfblk48 ==
  cfblk1 : Inport
  cfblk16 : Inport  Port=2
  cfblk10 : Subsystem
  cfblk11 : Subsystem
  cfblk12 : Subsystem
  cfblk13 : Subsystem
  cfblk14 : Subsystem
  cfblk15 : Subsystem
  cfblk{17..20} (4 alike) : Delay  SampleTime=1
  cfblk3 : simulink/Discrete/Transfer Fcn First Order  PoleZ=0.95  ICPrevOutput=0.0  DoSatur=off
  cfblk4 : Gain  Gain=[466896226.451821]
  cfblk5 : DotProduct  OutDataTypeStr=Inherit: Inherit via internal rule
  cfblk6 : Sin  TimeSource=Use external signal  SampleTime=0
  cfblk7 : Constant  Value=[644607202.314678]  SampleTime=1
  cfblk8 : Constant  Value=[707761513.034585]  SampleTime=1
  cfblk9 : Constant  Value=[-59422049.552913]  SampleTime=1
  cfblk2 : Outport
  wires:
  cfblk5/1 -> cfblk15/1(cfblk1), cfblk12/2(cfblk12)
  cfblk7/1 -> cfblk15/2(cfblk14)
  cfblk8/1 -> cfblk6/1
  cfblk10/1(cfblk2) -> cfblk13/1(cfblk1)
  cfblk6/1 -> cfblk10/1(cfblk1)
  cfblk16/1 -> cfblk14/1(cfblk1)
  cfblk3/1 -> cfblk4/1
  cfblk14/1(cfblk2) -> cfblk15/3(cfblk15)
  cfblk1/1 -> cfblk11/1(cfblk1)
  cfblk4/1 -> cfblk5/1, cfblk10/2(cfblk10)
  cfblk10/2(cfblk12) -> cfblk14/2(cfblk12)
  cfblk11/1(cfblk2) -> cfblk3/1, cfblk10/3(cfblk11)
  cfblk9/1 -> cfblk13/2(cfblk7)
  cfblk15/1(cfblk2) -> cfblk13/3(cfblk8)
  cfblk15/2(cfblk17) -> cfblk2/1
  cfblk13/2(cfblk9) -> cfblk12/1(cfblk1)
  cfblk13/1(cfblk2) -> cfblk17/1
  cfblk17/1 -> cfblk11/2(cfblk8)
  cfblk12/1(cfblk2) -> cfblk18/1
  cfblk18/1 -> cfblk5/2
  cfblk12/2(cfblk13) -> cfblk19/1
  cfblk19/1 -> cfblk15/4(cfblk16)
  cfblk12/3(cfblk14) -> cfblk20/1
  cfblk20/1 -> cfblk11/3(cfblk9)

== system sampleModel103/cfblk49 ==
  cfblk1 : Inport
  cfblk7 : Inport  Port=2
  cfblk8 : Inport  Port=3
  cfblk3 : UnitDelay  HasFrameUpgradeWarning=on
  cfblk4 : Signum
  cfblk5 : Sum  Inputs=|++
  cfblk6 : Constant  Value=[673121158.776354]  SampleTime=1
  cfblk9 : Delay  SampleTime=1
  cfblk2 : Outport
  wires:
  cfblk8/1 -> cfblk4/1
  cfblk1/1 -> cfblk2/1
  cfblk3/1 -> cfblk5/1
  cfblk7/1 -> cfblk5/2
  cfblk5/1 -> cfblk9/1
  cfblk9/1 -> cfblk3/1

== system sampleModel103/cfblk50 ==
  cfblk1 : Inport
  cfblk8 : Inport  Port=2
  cfblk3 : Delay  SampleTime=1
  cfblk4 : DiscreteTransferFcn  SampleTime=1
  cfblk5 : Sum  Inputs=|++
  cfblk6 : Sin  TimeSource=Use external signal  SampleTime=0
  cfblk7 : Constant  Value=[-929668017.490632]  SampleTime=1
  cfblk9 : Delay  SampleTime=1
  cfblk2 : Outport
  wires:
  cfblk8/1 -> cfblk5/1
  cfblk7/1 -> cfblk3/1
  cfblk6/1 -> cfblk5/2
  cfblk4/1 -> cfblk6/1
  cfblk1/1 -> cfblk2/1
  cfblk5/1 -> cfblk9/1
  cfblk9/1 -> cfblk4/1

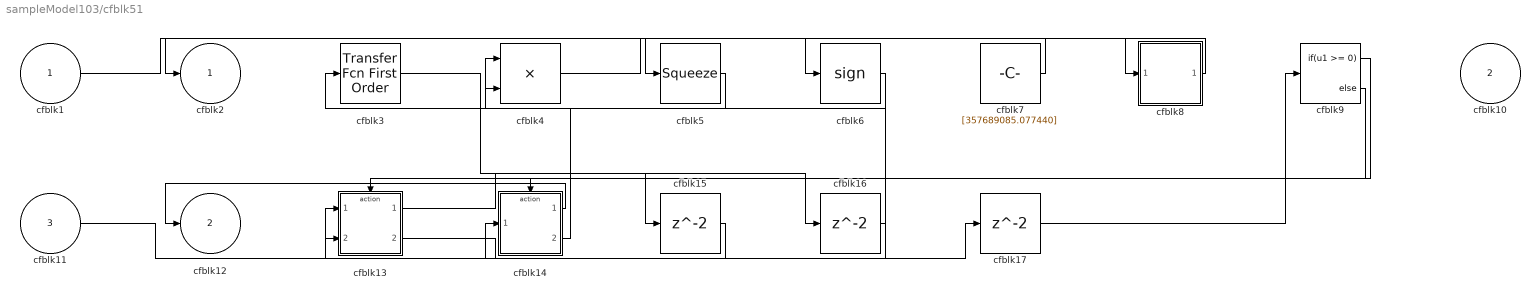
== system sampleModel103/cfblk51 ==
  cfblk1 : Inport
  cfblk10 : Inport  Port=2
  cfblk11 : Inport  Port=3
  cfblk13 : Subsystem  TreatAsAtomicUnit=on
  cfblk14 : Subsystem  TreatAsAtomicUnit=on
  cfblk15 : Delay  SampleTime=1
  cfblk16 : Delay  SampleTime=1
  cfblk17 : Delay  SampleTime=1
  cfblk3 : simulink/Discrete/Transfer Fcn First Order  PoleZ=0.95  ICPrevOutput=0.0  DoSatur=off
  cfblk4 : Product
  cfblk5 : Squeeze
  cfblk6 : Signum
  cfblk7 : Constant  Value=[357689085.077440]  SampleTime=1
  cfblk8 : Subsystem
  cfblk9 : If  IfExpression=u1 >= 0  SampleTime=1
  cfblk2 : Outport
  cfblk12 : Outport  Port=2
  wires:
  cfblk8/1(cfblk2) -> cfblk5/1
  cfblk14/1(cfblk2) -> cfblk12/1
  cfblk5/1 -> cfblk3/1
  cfblk11/1 -> cfblk13/1(cfblk1)
  cfblk6/1 -> cfblk14/1(cfblk1)
  cfblk7/1 -> cfblk2/1
  cfblk14/2(cfblk8) -> cfblk4/1
  cfblk1/1 -> cfblk6/1
  cfblk4/1 -> cfblk8/1(cfblk1)
  cfblk9/1 -> cfblk13/Action
  cfblk9/2 -> cfblk14/Action
  cfblk3/1 -> cfblk15/1
  cfblk15/1 -> cfblk13/2(cfblk11)
  cfblk13/1(cfblk2) -> cfblk16/1
  cfblk16/1 -> cfblk4/2
  cfblk13/2(cfblk12) -> cfblk17/1
  cfblk17/1 -> cfblk9/1

== system sampleModel103/cfblk53 ==
  cfblk1 : Inport
  cfblk6 : Inport  Port=2
  Action Port : ActionPort  ActionPortLabel=if(u1 >= 0)
  cfblk3 : DiscreteStateSpace  SampleTime=-1
  cfblk4 : Reshape
  cfblk5 : Subsystem
  cfblk2 : Outport
  cfblk7 : Outport  Port=2
  wires:
  cfblk1/1 -> cfblk4/1, cfblk5/2(cfblk12)
  cfblk4/1 -> cfblk3/1
  cfblk3/1 -> cfblk5/1(cfblk1), cfblk5/3(cfblk13)
  cfblk6/1 -> cfblk7/1, cfblk5/4(cfblk14), cfblk5/5(cfblk15)
  cfblk5/1(cfblk2) -> cfblk2/1

== system sampleModel103/cfblk54 ==
  cfblk1 : Inport
  cfblk7 : Inport  Port=2
  Action Port : ActionPort  ActionPortLabel=else
  cfblk10 : Delay
  cfblk3 : Delay  DelayLengthSource=Input port
      settings: InputPortMap=u0,p1
  cfblk4 : Trigonometry
  cfblk5 : Constant  Value=[-392594834.269827]  SampleTime=1
  cfblk6 : Subsystem
  cfblk2 : Outport
  cfblk8 : Outport  Port=2
  cfblk9 : Outport  Port=3
  wires:
  cfblk1/1 -> cfblk3/1
  cfblk7/1 -> cfblk3/2
  cfblk5/1 -> cfblk9/1, cfblk6/3(cfblk12)
  cfblk6/1(cfblk2) -> cfblk2/1
  cfblk6/2(cfblk13) -> cfblk8/1, cfblk4/1
  cfblk3/1 -> cfblk6/2(cfblk11)
  cfblk4/1 -> cfblk10/1
  cfblk10/1 -> cfblk6/1(cfblk1)

== system sampleModel103/cfblk40/cfblk8 ==
  cfblk1 : Inport
  cfblk11 : Inport  Port=2
  cfblk12 : Inport  Port=3
  cfblk10 : Constant  Value=[-256533590.078748]  SampleTime=1
  cfblk3 : simulink/Discrete/Transfer Fcn Lead or Lag  PoleZ=0.95  ZeroZ=0.75  ICPrevOutput=0.0  ICPrevInput=0.0  DoSatur=off
  cfblk4 : DiscreteTransferFcn  SampleTime=1
  cfblk5 : simulink/Math Operations/Slider Gain  gain=1  low=0  high=2
  cfblk6 : Signum
  cfblk7 : UnaryMinus
  cfblk8 : Product  Inputs=**
  cfblk9 : Constant  Value=[42384859.486859]  SampleTime=1
  cfblk2 : Outport
  wires:
  cfblk1/1 -> cfblk5/1
  cfblk3/1 -> cfblk7/1
  cfblk12/1 -> cfblk6/1
  cfblk11/1 -> cfblk8/1
  cfblk9/1 -> cfblk2/1
  cfblk10/1 -> cfblk3/1
  cfblk4/1 -> cfblk8/2
  cfblk5/1 -> cfblk4/1

== system sampleModel103/cfblk40/cfblk9 ==
  cfblk1 : Inport
  cfblk8 : Inport  Port=2
  cfblk3 : Delay  DelayLengthSource=Input port  SampleTime=1
      settings: InputPortMap=u0,p1
  cfblk4 : DiscreteZeroPole  Poles=[0 0.5]  Gain=1
  cfblk5 : Reshape
  cfblk6 : Rounding
  cfblk7 : Math  Operator=log10
  cfblk2 : Outport
  wires:
  cfblk1/1 -> cfblk5/1
  cfblk3/1 -> cfblk2/1
  cfblk8/1 -> cfblk6/1
  cfblk5/1 -> cfblk7/1
  cfblk7/1 -> cfblk4/1
  cfblk6/1 -> cfblk3/1
  cfblk4/1 -> cfblk3/2

== system sampleModel103/cfblk41/cfblk10 ==
  cfblk1 : Inport
  cfblk14 : Inport  Port=2
  cfblk10 : Constant  Value=[-45251306.932969]  SampleTime=1
  cfblk11 : Constant  Value=[-417889505.493051]  SampleTime=1
  cfblk12 : Constant  Value=[-762804193.727089]  SampleTime=1
  cfblk13 : Constant  Value=[-417496993.322412]  SampleTime=1
  cfblk3 : UnitDelay  HasFrameUpgradeWarning=on
  cfblk4 : simulink/Discrete/Transfer Fcn First Order  PoleZ=0.95  ICPrevOutput=0.0  DoSatur=off
  cfblk5 : DiscreteZeroPole  Poles=[0 0.5]  Gain=1
  cfblk6 : DiscreteZeroPole  Poles=[0 0.5]  Gain=1
  cfblk7 : Product
  cfblk8 : Sqrt
  cfblk9 : Abs  SaturateOnIntegerOverflow=off
  cfblk2 : Outport
  cfblk15 : Outport  Port=2
  cfblk16 : Outport  Port=3
  wires:
  cfblk14/1 -> cfblk16/1
  cfblk6/1 -> cfblk2/1
  cfblk12/1 -> cfblk6/1
  cfblk11/1 -> cfblk5/1
  cfblk5/1 -> cfblk3/1
  cfblk4/1 -> cfblk8/1
  cfblk1/1 -> cfblk15/1
  cfblk13/1 -> cfblk7/1
  cfblk10/1 -> cfblk9/1
  cfblk3/1 -> cfblk4/1
  cfblk8/1 -> cfblk7/2

== system sampleModel103/cfblk41/cfblk11 ==
  cfblk1 : Inport
  cfblk6 : Inport  Port=2
  cfblk3 : DiscreteFilter  SampleTime=1
  cfblk4 : DiscreteFilter  SampleTime=1
  cfblk5 : simulink/Discrete/Tapped Delay  vinit=0.0  samptime=-1  NumDelays=1  DelayOrder=Oldest  includeCurrent=off
  cfblk2 : Outport
  cfblk7 : Outport  Port=2
  wires:
  cfblk5/1 -> cfblk7/1, cfblk3/1
  cfblk1/1 -> cfblk2/1
  cfblk6/1 -> cfblk4/1
  cfblk4/1 -> cfblk5/1

== system sampleModel103/cfblk41/cfblk12 ==
  cfblk1 : Inport
  cfblk10 : Inport  Port=2
  cfblk11 : Inport  Port=3
  cfblk3 : DiscreteFir  SampleTime=1
  cfblk4 : simulink/Discrete/Transfer Fcn Lead or Lag  PoleZ=0.95  ZeroZ=0.75  ICPrevOutput=0.0  ICPrevInput=0.0  DoSatur=off
  cfblk5 : DiscreteTransferFcn  SampleTime=1
  cfblk6 : simulink/Discrete/Tapped Delay  vinit=0.0  samptime=-1  NumDelays=1  DelayOrder=Oldest  includeCurrent=off
  cfblk7 : UnaryMinus
  cfblk8 : Signum
  cfblk9 : Constant  Value=[-533592757.000974]  SampleTime=1
  cfblk2 : Outport
  cfblk12 : Outport  Port=2
  wires:
  cfblk9/1 -> cfblk4/1
  cfblk8/1 -> cfblk3/1
  cfblk4/1 -> cfblk5/1
  cfblk3/1 -> cfblk7/1
  cfblk7/1 -> cfblk12/1
  cfblk1/1 -> cfblk8/1
  cfblk10/1 -> cfblk6/1
  cfblk11/1 -> cfblk2/1

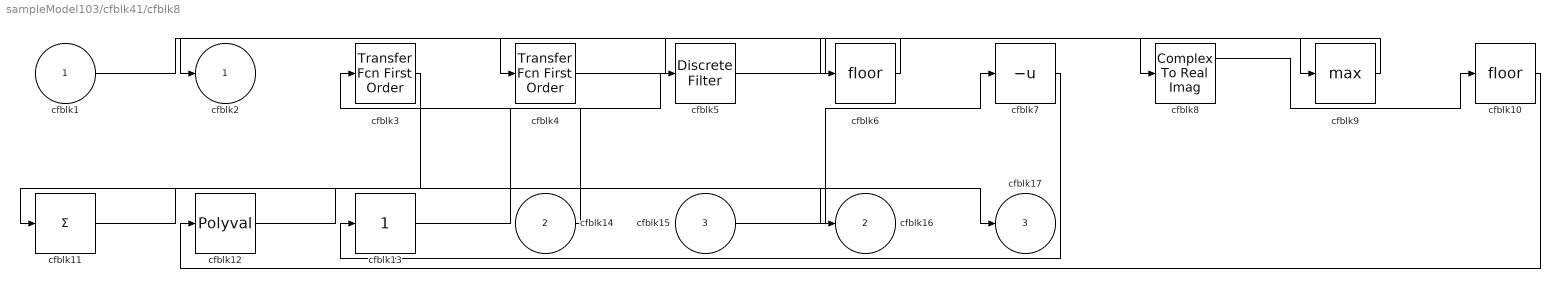
== system sampleModel103/cfblk41/cfblk8 ==
  cfblk1 : Inport
  cfblk14 : Inport  Port=2
  cfblk15 : Inport  Port=3
  cfblk10 : Rounding
  cfblk11 : Sum  Inputs=+
  cfblk12 : Polyval  Coefs=[ +2.081618890e-019, -1.441693666e-014, +4.719686976e-010, -8.536869453e-006, +1.621573104e-001, -8.087801117e+001 ]
  cfblk13 : simulink/Math Operations/Slider Gain  gain=1  low=0  high=2
  cfblk3 : simulink/Discrete/Transfer Fcn First Order  PoleZ=0.95  ICPrevOutput=0.0  DoSatur=off
  cfblk4 : simulink/Discrete/Transfer Fcn First Order  PoleZ=0.95  ICPrevOutput=0.0  DoSatur=off
  cfblk5 : DiscreteFilter  SampleTime=1
  cfblk6 : Rounding
  cfblk7 : UnaryMinus
  cfblk8 : ComplexToRealImag
  cfblk9 : MinMax  Function=max
  cfblk2 : Outport
  cfblk16 : Outport  Port=2
  cfblk17 : Outport  Port=3
  wires:
  cfblk6/1 -> cfblk2/1
  cfblk15/1 -> cfblk7/1
  cfblk7/1 -> cfblk13/1
  cfblk14/1 -> cfblk3/1
  cfblk5/1 -> cfblk8/1
  cfblk10/1 -> cfblk12/1
  cfblk3/1 -> cfblk11/1
  cfblk11/1 -> cfblk17/1
  cfblk4/1 -> cfblk9/1
  cfblk1/1 -> cfblk4/1
  cfblk13/1 -> cfblk5/1
  cfblk8/1 -> cfblk10/1
  cfblk12/1 -> cfblk16/1
  cfblk9/1 -> cfblk6/1

== system sampleModel103/cfblk41/cfblk9 ==
  cfblk1 : Inport
  cfblk6 : Inport  Port=2
  cfblk7 : Inport  Port=3
  cfblk8 : Inport  Port=4
  cfblk3 : DiscreteZeroPole  Poles=[0 0.5]  Gain=1
  cfblk4 : Constant  Value=[518432608.303579]  SampleTime=1
  cfblk5 : Constant  Value=[-220236754.760621]  SampleTime=1
  cfblk2 : Outport
  wires:
  cfblk4/1 -> cfblk3/1
  cfblk8/1 -> cfblk2/1

== system sampleModel103/cfblk42/cfblk7 ==
  cfblk1 : Inport
  cfblk7 : Inport  Port=2
  cfblk3 : DiscreteFilter  SampleTime=1
  cfblk4 : DotProduct  OutDataTypeStr=Inherit: Inherit via internal rule
  cfblk5 : Rounding
  cfblk6 : Constant  Value=[-915522887.961784]  SampleTime=1
  cfblk2 : Outport
  cfblk8 : Outport  Port=2
  wires:
  cfblk3/1 -> cfblk5/1
  cfblk1/1 -> cfblk3/1
  cfblk7/1 -> cfblk2/1
  cfblk4/1 -> cfblk8/1
  cfblk5/1 -> cfblk4/1
  cfblk6/1 -> cfblk4/2

== system sampleModel103/cfblk42/cfblk8 ==
  cfblk1 : Inport
  cfblk3 : DiscreteFir  SampleTime=1
  cfblk4 : DiscreteZeroPole  Poles=[0 0.5]  Gain=1
  cfblk5 : UnaryMinus
  cfblk6 : Trigonometry
  cfblk7 : Rounding
  cfblk2 : Outport
  cfblk8 : Outport  Port=2
  wires:
  cfblk3/1 -> cfblk4/1, cfblk2/1
  cfblk1/1 -> cfblk6/1
  cfblk6/1 -> cfblk5/1
  cfblk5/1 -> cfblk7/1
  cfblk4/1 -> cfblk8/1
  cfblk7/1 -> cfblk3/1

== system sampleModel103/cfblk42/cfblk9 ==
  cfblk1 : Inport
  cfblk5 : Inport  Port=2
  cfblk3 : UnaryMinus
  cfblk4 : DotProduct  OutDataTypeStr=Inherit: Inherit via internal rule
  cfblk2 : Outport
  cfblk6 : Outport  Port=2
  cfblk7 : Outport  Port=3
  wires:
  cfblk3/1 -> cfblk2/1
  cfblk1/1 -> cfblk4/1, cfblk3/1
  cfblk5/1 -> cfblk4/2, cfblk6/1
  cfblk4/1 -> cfblk7/1

== system sampleModel103/cfblk43/cfblk8 ==
  cfblk1 : Inport
  cfblk3 : Delay  DelayLengthSource=Input port  SampleTime=1
      settings: InputPortMap=u0,p1
  cfblk4 : slpidlib/PID Controller  Controller=PID  Form=Parallel  TimeDomain=Discrete-time  UseExternalTs=off  SampleTime=1  IntegratorMethod=Forward Euler  FilterMethod=Forward Euler  ControllerParametersSource=internal  P=1  I=1  UseKiTs=off  D=0  N=100  UseFilter=on  TunerSelectOption=Transfer Function Based (PID Tuner App)  InitialConditionSource=internal  InitialConditionForIntegrator=0  InitialConditionForFilter=0  DifferentiatorICPrevScaledInput=0  ExternalReset=none  TrackingMode=off  Kt=1  LimitOutput=off  SatLimitsSource=internal  UpperSaturationLimit=inf  LowerSaturationLimit=-inf  LinearizeAsGain=off  AntiWindupMode=none  Kb=1  LimitIntegrator=off  UpperIntegratorSaturationLimit=inf  LowerIntegratorSaturationLimit=-inf  POutMin=[]  POutMax=[]  IOutMin=[]  IOutMax=[]  DOutMin=[]  DOutMax=[]  NOutMin=[]  NOutMax=[]  SumOutMin=[]  SumOutMax=[]  SaturationOutMin=[]  SaturationOutMax=[]  PParamMin=[]  PParamMax=[]  IParamMin=[]  IParamMax=[]  DParamMin=[]  DParamMax=[]  NParamMin=[]  NParamMax=[]  KbParamMin=[]  KbParamMax=[]  KtParamMin=[]  KtParamMax=[]  KbOutMin=[]  KbOutMax=[]  KtOutMin=[]  KtOutMax=[]  IntegratorOutMin=[]  IntegratorOutMax=[]  FilterOutMin=[]  FilterOutMax=[]  SumI1OutMin=[]  SumI1OutMax=[]  SumI2OutMin=[]  SumI2OutMax=[]  SumI3OutMin=[]  SumI3OutMax=[]  SumI4OutMin=[]  SumI4OutMax=[]  SumDOutMin=[]  SumDOutMax=[]  DifferentiatorOutMin=[]  DifferentiatorOutMax=[]  FilterDiffOutCoefMin=[]  FilterDiffOutCoefMax=[]  ReciprocalOutMin=[]  ReciprocalOutMax=[]  SumDenOutMin=[]  SumDenOutMax=[]  SumNumOutMin=[]  SumNumOutMax=[]  DivideOutMin=[]  DivideOutMax=[]  UdiffTsProdOutMin=[]  UdiffTsProdOutMax=[]  NTsProdOutMin=[]  NTsProdOutMax=[]  UintegralTsProdOutMin=[]  UintegralTsProdOutMax=[]  UngainTsProdOutMin=[]  UngainTsProdOutMax=[]  ClampingZeroOutDataTypeStr=Inherit: Inherit via back propagation  ClampingZeroOutMin=[]  ClampingZeroOutMax=[]  FilterDenConstantOutDataTypeStr=Inherit: Inherit via back propagation  FilterDenConstantOutMin=[]  FilterDenConstantOutMax=[]  PCopyOutDataTypeStr=Inherit: Inherit via back propagation  PCopyOutMin=[]  PCopyOutMax=[]  NCopyOutDataTypeStr=Inherit: Inherit via back propagation  NCopyOutMin=[]  NCopyOutMax=[]  IntegratorContinuousStateAttributes=''  IntegratorStateMustResolveToSignalObject=off  IntegratorRTWStateStorageClass=Auto  FilterContinuousStateAttributes=''  FilterStateMustResolveToSignalObject=off  FilterRTWStateStorageClass=Auto  ParallelPVariant=InternalParameters  IdealPVariant=Disabled  IVariant=InternalParameters  DVariant=InternalParameters  IntegratorVariant=Discrete  SatVariant=Disabled  AWVariant=Passthrough  PCopyVariant=Disabled  TRVariant=Disabled  FdbkBlocksVariant=Forward  IdealPFdbkVariant=Disabled  SatFdbkVariant=Disabled  DerivativeFilterVariant=ForwardEulerFilter  NVariant=InternalParameters  NCopyVariant=Disabled  FilterICVariant=InternalICsFilter  IntegratorICVariant=InternalICs  ExternalResetVariant=Disabled  TRSumVariant=Passthrough  SumFdbkVariant=Disabled  SumVariant=Sum_PID  TsampFilterVariant=InternalTs  TsampNgainVariant=Passthrough  TsampIntegralVariant=Disabled_SignalSpec  ExternalSaturationOutDataTypeStr=Inherit: Same as second input
      settings: LibrarySourceBlock=simulink/Discrete/Discrete PID Controller
  cfblk5 : slpidlib/PID Controller (2DOF)  Controller=PID  Form=Parallel  TimeDomain=Discrete-time  UseExternalTs=off  SampleTime=1  IntegratorMethod=Forward Euler  FilterMethod=Forward Euler  ControllerParametersSource=internal  P=1  I=1  UseKiTs=off  D=0  N=100  UseFilter=on  b=1  c=1  TunerSelectOption=Transfer Function Based (PID Tuner App)  InitialConditionSource=internal  InitialConditionForIntegrator=0  InitialConditionForFilter=0  DifferentiatorICPrevScaledInput=0  ExternalReset=none  TrackingMode=off  Kt=1  LimitOutput=off  SatLimitsSource=internal  UpperSaturationLimit=inf  LowerSaturationLimit=-inf  LinearizeAsGain=off  AntiWindupMode=none  Kb=1  LimitIntegrator=off  UpperIntegratorSaturationLimit=inf  LowerIntegratorSaturationLimit=-inf  POutMin=[]  POutMax=[]  IOutMin=[]  IOutMax=[]  DOutMin=[]  DOutMax=[]  NOutMin=[]  NOutMax=[]  bOutMin=[]  bOutMax=[]  cOutMin=[]  cOutMax=[]  SumOutMin=[]  SumOutMax=[]  SaturationOutMin=[]  SaturationOutMax=[]  PParamMin=[]  PParamMax=[]  IParamMin=[]  IParamMax=[]  DParamMin=[]  DParamMax=[]  NParamMin=[]  NParamMax=[]  bParamMin=[]  bParamMax=[]  cParamMin=[]  cParamMax=[]  KbParamMin=[]  KbParamMax=[]  KtParamMin=[]  KtParamMax=[]  KbOutMin=[]  KbOutMax=[]  KtOutMin=[]  KtOutMax=[]  IntegratorOutMin=[]  IntegratorOutMax=[]  FilterOutMin=[]  FilterOutMax=[]  SumI1OutMin=[]  SumI1OutMax=[]  SumI2OutMin=[]  SumI2OutMax=[]  SumI3OutMin=[]  SumI3OutMax=[]  SumI4OutMin=[]  SumI4OutMax=[]  SumDOutMin=[]  SumDOutMax=[]  Sum1OutMin=[]  Sum1OutMax=[]  Sum2OutMin=[]  Sum2OutMax=[]  Sum3OutMin=[]  Sum3OutMax=[]  DifferentiatorOutMin=[]  DifferentiatorOutMax=[]  FilterDiffOutCoefMin=[]  FilterDiffOutCoefMax=[]  ReciprocalOutMin=[]  ReciprocalOutMax=[]  SumDenOutMin=[]  SumDenOutMax=[]  SumNumOutMin=[]  SumNumOutMax=[]  DivideOutMin=[]  DivideOutMax=[]  UdiffTsProdOutMin=[]  UdiffTsProdOutMax=[]  NTsProdOutMin=[]  NTsProdOutMax=[]  UintegralTsProdOutMin=[]  UintegralTsProdOutMax=[]  UngainTsProdOutMin=[]  UngainTsProdOutMax=[]  ClampingZeroOutDataTypeStr=Inherit: Inherit via back propagation  ClampingZeroOutMin=[]  ClampingZeroOutMax=[]  FilterDenConstantOutDataTypeStr=Inherit: Inherit via back propagation  FilterDenConstantOutMin=[]  FilterDenConstantOutMax=[]  PCopyOutDataTypeStr=Inherit: Inherit via back propagation  PCopyOutMin=[]  PCopyOutMax=[]  NCopyOutDataTypeStr=Inherit: Inherit via back propagation  NCopyOutMin=[]  NCopyOutMax=[]  IntegratorContinuousStateAttributes=''  IntegratorStateMustResolveToSignalObject=off  IntegratorRTWStateStorageClass=Auto  FilterContinuousStateAttributes=''  FilterStateMustResolveToSignalObject=off  FilterRTWStateStorageClass=Auto  ParallelPVariant=InternalParameters  IdealPVariant=Disabled  IVariant=InternalParameters  DVariant=InternalParameters  bVariant=InternalParameters  cVariant=InternalParameters  IntegratorVariant=Discrete  SatVariant=Disabled  AWVariant=Passthrough  PCopyVariant=Disabled  TRVariant=Disabled  FdbkBlocksVariant=Forward  IdealPFdbkVariant=Disabled  SatFdbkVariant=Disabled  DerivativeFilterVariant=ForwardEulerFilter  NVariant=InternalParameters  NCopyVariant=Disabled  FilterICVariant=InternalICsFilter  IntegratorICVariant=InternalICs  ExternalResetVariant=Disabled  TRSumVariant=Passthrough  SumFdbkVariant=Disabled  SumVariant=Sum_PID  TsampFilterVariant=InternalTs  TsampNgainVariant=Passthrough  TsampIntegralVariant=Disabled_SignalSpec  ExternalSaturationOutDataTypeStr=Inherit: Same as second input
      settings: LibrarySourceBlock=simulink/Discrete/Discrete PID Controller (2DOF)
  cfblk6 : slpidlib/PID Controller  Controller=PID  Form=Parallel  TimeDomain=Discrete-time  UseExternalTs=off  SampleTime=1  IntegratorMethod=Forward Euler  FilterMethod=Forward Euler  ControllerParametersSource=internal  P=1  I=1  UseKiTs=off  D=0  N=100  UseFilter=on  TunerSelectOption=Transfer Function Based (PID Tuner App)  InitialConditionSource=internal  InitialConditionForIntegrator=0  InitialConditionForFilter=0  DifferentiatorICPrevScaledInput=0  ExternalReset=none  TrackingMode=off  Kt=1  LimitOutput=off  SatLimitsSource=internal  UpperSaturationLimit=inf  LowerSaturationLimit=-inf  LinearizeAsGain=off  AntiWindupMode=none  Kb=1  LimitIntegrator=off  UpperIntegratorSaturationLimit=inf  LowerIntegratorSaturationLimit=-inf  POutMin=[]  POutMax=[]  IOutMin=[]  IOutMax=[]  DOutMin=[]  DOutMax=[]  NOutMin=[]  NOutMax=[]  SumOutMin=[]  SumOutMax=[]  SaturationOutMin=[]  SaturationOutMax=[]  PParamMin=[]  PParamMax=[]  IParamMin=[]  IParamMax=[]  DParamMin=[]  DParamMax=[]  NParamMin=[]  NParamMax=[]  KbParamMin=[]  KbParamMax=[]  KtParamMin=[]  KtParamMax=[]  KbOutMin=[]  KbOutMax=[]  KtOutMin=[]  KtOutMax=[]  IntegratorOutMin=[]  IntegratorOutMax=[]  FilterOutMin=[]  FilterOutMax=[]  SumI1OutMin=[]  SumI1OutMax=[]  SumI2OutMin=[]  SumI2OutMax=[]  SumI3OutMin=[]  SumI3OutMax=[]  SumI4OutMin=[]  SumI4OutMax=[]  SumDOutMin=[]  SumDOutMax=[]  DifferentiatorOutMin=[]  DifferentiatorOutMax=[]  FilterDiffOutCoefMin=[]  FilterDiffOutCoefMax=[]  ReciprocalOutMin=[]  ReciprocalOutMax=[]  SumDenOutMin=[]  SumDenOutMax=[]  SumNumOutMin=[]  SumNumOutMax=[]  DivideOutMin=[]  DivideOutMax=[]  UdiffTsProdOutMin=[]  UdiffTsProdOutMax=[]  NTsProdOutMin=[]  NTsProdOutMax=[]  UintegralTsProdOutMin=[]  UintegralTsProdOutMax=[]  UngainTsProdOutMin=[]  UngainTsProdOutMax=[]  ClampingZeroOutDataTypeStr=Inherit: Inherit via back propagation  ClampingZeroOutMin=[]  ClampingZeroOutMax=[]  FilterDenConstantOutDataTypeStr=Inherit: Inherit via back propagation  FilterDenConstantOutMin=[]  FilterDenConstantOutMax=[]  PCopyOutDataTypeStr=Inherit: Inherit via back propagation  PCopyOutMin=[]  PCopyOutMax=[]  NCopyOutDataTypeStr=Inherit: Inherit via back propagation  NCopyOutMin=[]  NCopyOutMax=[]  IntegratorContinuousStateAttributes=''  IntegratorStateMustResolveToSignalObject=off  IntegratorRTWStateStorageClass=Auto  FilterContinuousStateAttributes=''  FilterStateMustResolveToSignalObject=off  FilterRTWStateStorageClass=Auto  ParallelPVariant=InternalParameters  IdealPVariant=Disabled  IVariant=InternalParameters  DVariant=InternalParameters  IntegratorVariant=Discrete  SatVariant=Disabled  AWVariant=Passthrough  PCopyVariant=Disabled  TRVariant=Disabled  FdbkBlocksVariant=Forward  IdealPFdbkVariant=Disabled  SatFdbkVariant=Disabled  DerivativeFilterVariant=ForwardEulerFilter  NVariant=InternalParameters  NCopyVariant=Disabled  FilterICVariant=InternalICsFilter  IntegratorICVariant=InternalICs  ExternalResetVariant=Disabled  TRSumVariant=Passthrough  SumFdbkVariant=Disabled  SumVariant=Sum_PID  TsampFilterVariant=InternalTs  TsampNgainVariant=Passthrough  TsampIntegralVariant=Disabled_SignalSpec  ExternalSaturationOutDataTypeStr=Inherit: Same as second input
      settings: LibrarySourceBlock=simulink/Discrete/Discrete PID Controller
  cfblk7 : ComplexToMagnitudeAngle
  cfblk8 : Delay  SampleTime=1
  cfblk9 : Delay  SampleTime=1
  cfblk2 : Outport
  wires:
  cfblk4/1 -> cfblk7/1
  cfblk3/1 -> cfblk6/1
  cfblk1/1 -> cfblk2/1
  cfblk6/1 -> cfblk4/1, cfblk5/1
  cfblk7/2 -> cfblk5/2, cfblk9/1
  cfblk7/1 -> cfblk8/1
  cfblk8/1 -> cfblk3/1
  cfblk9/1 -> cfblk3/2

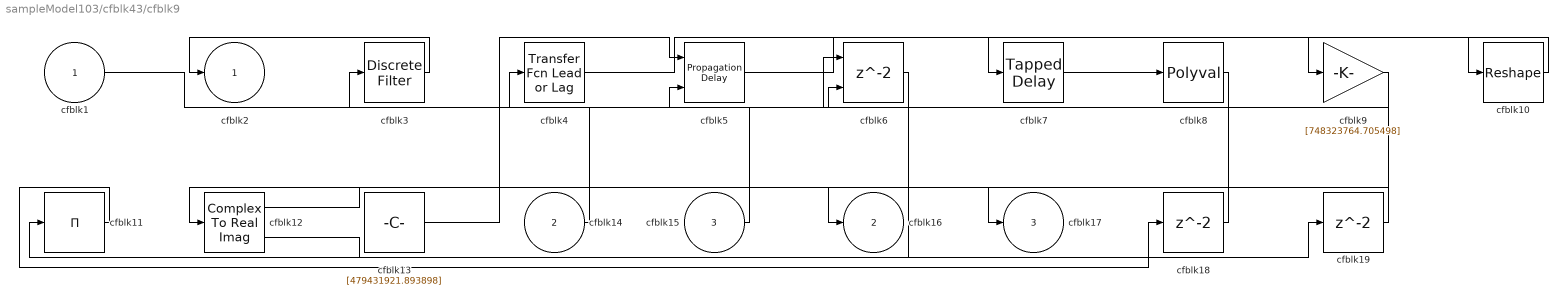
== system sampleModel103/cfblk43/cfblk9 ==
  cfblk1 : Inport
  cfblk14 : Inport  Port=2
  cfblk15 : Inport  Port=3
  cfblk10 : Reshape
  cfblk11 : Product  Inputs=*
  cfblk12 : ComplexToRealImag
  cfblk13 : Constant  Value=[479431921.893898]  SampleTime=1
  cfblk18 : Delay  SampleTime=1
  cfblk19 : Delay  SampleTime=1
  cfblk3 : DiscreteFilter  SampleTime=1
  cfblk4 : simulink/Discrete/Transfer Fcn Lead or Lag  PoleZ=0.95  ZeroZ=0.75  ICPrevOutput=0.0  ICPrevInput=0.0  DoSatur=off
  cfblk5 : PropagationDelay  SampleTime=1
  cfblk6 : Delay  ShowEnablePort=on  SampleTime=1
      settings: InputPortMap=u0,e6
  cfblk7 : simulink/Discrete/Tapped Delay  vinit=0.0  samptime=-1  NumDelays=1  DelayOrder=Oldest  includeCurrent=off
  cfblk8 : Polyval  Coefs=[ +2.081618890e-019, -1.441693666e-014, +4.719686976e-010, -8.536869453e-006, +1.621573104e-001, -8.087801117e+001 ]
  cfblk9 : Gain  Gain=[748323764.705498]
  cfblk2 : Outport
  cfblk16 : Outport  Port=2
  cfblk17 : Outport  Port=3
  wires:
  cfblk4/1 -> cfblk7/1
  cfblk15/1 -> cfblk4/1
  cfblk10/1 -> cfblk9/1
  cfblk3/1 -> cfblk2/1
  cfblk8/1 -> cfblk17/1
  cfblk6/1 -> cfblk11/1
  cfblk7/1 -> cfblk8/1
  cfblk13/1 -> cfblk5/1
  cfblk5/1 -> cfblk10/1
  cfblk14/1 -> cfblk3/1
  cfblk12/1 -> cfblk16/1
  cfblk9/1 -> cfblk12/1
  cfblk1/1 -> cfblk6/2
  cfblk11/1 -> cfblk18/1
  cfblk18/1 -> cfblk6/1
  cfblk12/2 -> cfblk19/1
  cfblk19/1 -> cfblk5/2

== system sampleModel103/cfblk44/cfblk10 ==
  cfblk1 : Inport
  cfblk11 : Inport  Port=2
  cfblk12 : Inport  Port=3
  cfblk13 : Inport  Port=4
  cfblk10 : Product  Inputs=*
  cfblk3 : DiscreteZeroPole  Poles=[0 0.5]  Gain=1
  cfblk4 : simulink/Discrete/Transfer Fcn First Order  PoleZ=0.95  ICPrevOutput=0.0  DoSatur=off
  cfblk5 : Delay  SampleTime=1
  cfblk6 : Sum  Inputs=|++
  cfblk7 : Math  Operator=log
  cfblk8 : Sum  Inputs=+-
  cfblk9 : DotProduct  OutDataTypeStr=Inherit: Inherit via internal rule
  cfblk2 : Outport
  wires:
  cfblk10/1 -> cfblk6/1
  cfblk1/1 -> cfblk3/1
  cfblk7/1 -> cfblk8/1
  cfblk6/1 -> cfblk9/1
  cfblk3/1 -> cfblk9/2
  cfblk8/1 -> cfblk6/2
  cfblk11/1 -> cfblk7/1
  cfblk13/1 -> cfblk5/1
  cfblk12/1 -> cfblk10/1
  cfblk4/1 -> cfblk2/1
  cfblk5/1 -> cfblk8/2
  cfblk9/1 -> cfblk4/1
